simulink model "End_eff_test_7"  (R2023b)
settings: Solver=VariableStepAuto  StartTime=0.0  StopTime=10.0  RelTol=1e-3
undefined symbols (not defined in the file or in its folder): Levenberg, Marquardt
libraries: simulink x3, robotcorelib x1, robotmaniplib x1
settings Model: Creator=apoorvauplap  LastModifiedBy=apoorvauplap
settings DataIOCC: ReturnWorkspaceOutputs=off

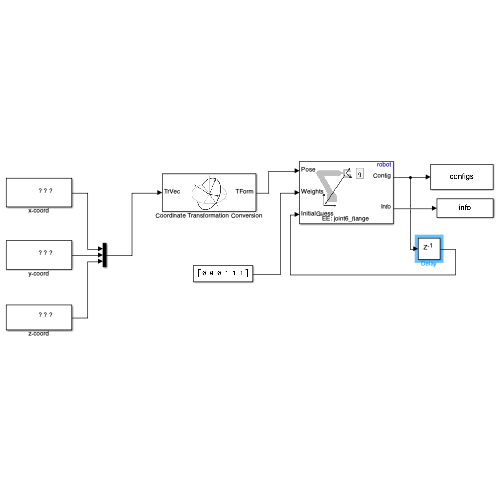
[thumbnail: Simulink's stored preview of the top-level diagram]
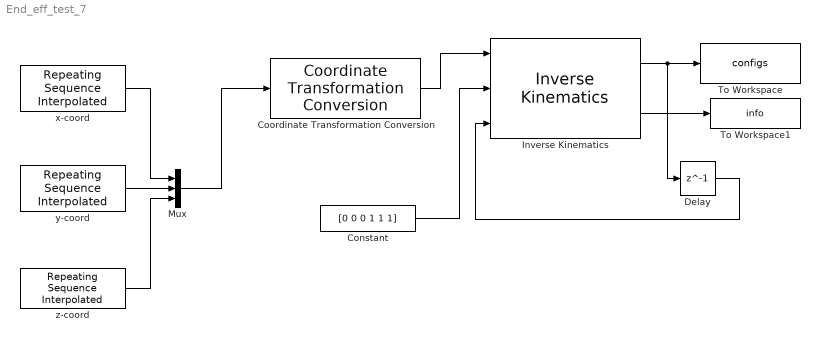
== system End_eff_test_7 ==
  Constant : Constant  Value=[0 0 0 1 1 1]
  Coordinate Transformation Conversion : robotcorelib/Coordinate Transformation Conversion  InputRepresentation=Translation Vector  InputEulerSequence=ZYX  ShowTrVecInputPort=on  OutputRepresentation=Homogeneous Transformation  OutputEulerSequence=ZYX  ShowTrVecOutputPort=on  SimulateUsing=Interpreted execution
  Delay : Delay  DelayLength=1  InitialCondition=zeros(6,1)
  Inverse Kinematics : robotmaniplib/Inverse Kinematics  RigidBodyTree=robot  EndEffector=joint6_flange  ShowInfo=on  SolverName=Levenberg-Marquardt  EnforceJointLimits=on  MaxIterations=1500  MaxTime=10  GradientTolerance=1e-7  SolutionTolerance=1e-6  StepTolerance=1e-14  ErrorChangeTolerance=1e-12  UseErrorDamping=on  DampingBias=0.0025  SimulateUsing=Interpreted execution
  Mux : Mux  Inputs=3
  To Workspace : ToWorkspace  VariableName=configs  SaveFormat=Timeseries  SampleTime=-1
  To Workspace1 : ToWorkspace  VariableName=info  SaveFormat=Timeseries  SampleTime=-1
  x-coord : simulink/Sources/Repeating Sequence Interpolated  OutValues=x  TimeValues=linspace(0,10,7)  LookUpMeth=Interpolation-Use End Values  tsamp=0.01  OutMin=[]  OutMax=[]  OutDataTypeStr=double  OutputDataTypeScalingMode=double  OutDataType=fixdt(0,8)  OutScaling=2^-10
  y-coord : simulink/Sources/Repeating Sequence Interpolated  OutValues=y  TimeValues=linspace(0,10,7)  LookUpMeth=Interpolation-Use End Values  tsamp=0.01  OutMin=[]  OutMax=[]  OutDataTypeStr=double  OutputDataTypeScalingMode=double  OutDataType=fixdt(0,8)  OutScaling=2^-10
  z-coord : simulink/Sources/Repeating Sequence Interpolated  OutValues=z  TimeValues=linspace(0,10,7)  LookUpMeth=Interpolation-Use End Values  tsamp=0.01  OutMin=[]  OutMax=[]  OutDataTypeStr=double  OutputDataTypeScalingMode=double  OutDataType=fixdt(0,8)  OutScaling=2^-10
  wires:
  Constant/1 -> Inverse Kinematics/2
  Coordinate Transformation Conversion/1 -> Inverse Kinematics/1
  Inverse Kinematics/1 -> Delay/1, To Workspace/1
  Inverse Kinematics/2 -> To Workspace1/1
  Delay/1 -> Inverse Kinematics/3
  Mux/1 -> Coordinate Transformation Conversion/1
  z-coord/1 -> Mux/3
  y-coord/1 -> Mux/2
  x-coord/1 -> Mux/1
